simulink model "FinalProject"  (R2023b)
settings: Solver=VariableStepAuto  StartTime=0.0  StopTime=inf  RelTol=1e-3
libraries: instrumentseriallib x3
settings Model: Creator=Ngsanchong  LastModifiedBy=Ngsanchong

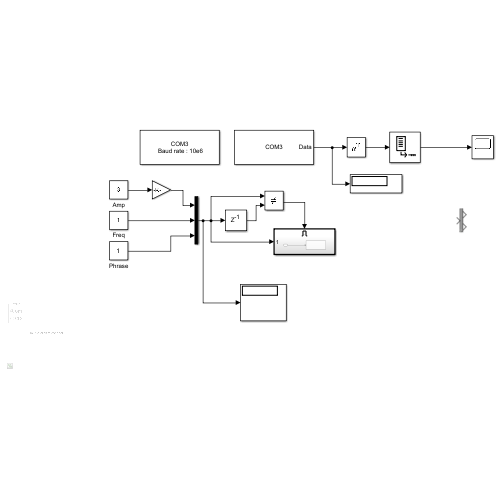
[thumbnail: Simulink's stored preview of the top-level diagram]
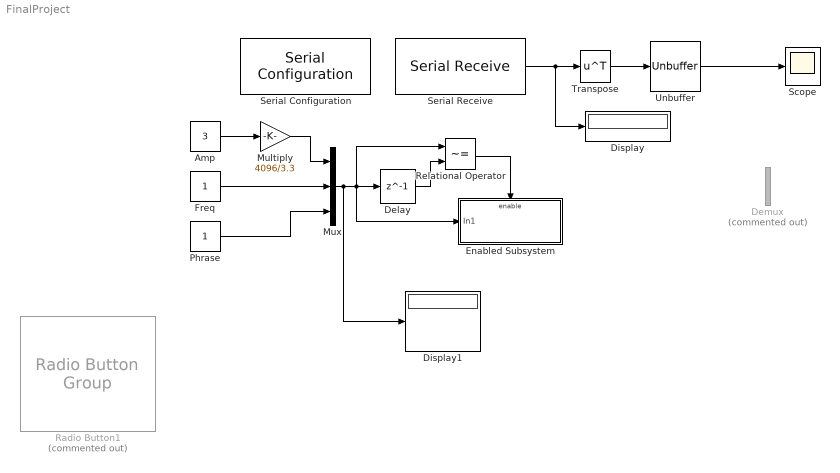
== system FinalProject ==
  Amp : Constant  Value=3  OutDataTypeStr=double
  Delay : Delay  DelayLength=1
  Demux : Demux  Commented=on  Outputs=2
  Display : Display
  Display1 : Display
  Enabled Subsystem : Subsystem  TreatAsAtomicUnit=on
  Freq : Constant  OutDataTypeStr=uint16
  Multiply : Gain  Gain=4096/3.3  OutMin=[0]  OutMax=[4096]  OutDataTypeStr=uint16
  Mux : Mux  Inputs=3
  Phrase : Constant  OutDataTypeStr=uint16
  Radio Button1 : RadioButtonGroup  Commented=on  ButtonGroupName=Group
      settings: Values={{'Ch1', 'Ch2'}, [0 1]}
  Relational Operator : RelationalOperator  Operator=~=  OutDataTypeStr=boolean  RndMeth=Simplest  InputSameDT=off
  Scope : Scope
  Serial Configuration : instrumentseriallib/Serial Configuration  Priority=-200000  PortSel=COM3  Port=COM3  ComPort=COM3  BaudRate=10e6  DataBits=8  Parity=none  StopBits=1  ByteOrder=little-endian  FlowControl=none  Timeout=10  SimulateUsing=Interpreted execution  BlockInModel=on  aMode=1
      settings: LibrarySourceBlock=c2000lib/Host Communication/Serial Configuration
  Serial Receive : instrumentseriallib/Serial Receive  Priority=1  PortSel=COM3  Port=COM3  ComPort=COM3  DataType=int16  SaveDataType=uint8  ToggleHeader=off  Header=[]  ToggleTerminator=off  Terminator=<none>  CustomTerminator=[]  InputFormat=Column major  ToggleDataSize=on  DataSize=[1 2000]  EnableBlockingMode=on  ActionDataUnavailable=Output last received value  ActionWhenDataUnavailable=Output last received value  CustomValue=0  SampleTime=0.02  SimulateUsing=Interpreted execution  BlockInModel=on  aMode=1
      settings: LibrarySourceBlock=c2000lib/Host Communication/Serial Receive
  Transpose : Math  Operator=transpose
  Unbuffer : Unbuffer
  wires:
  Serial Receive/1 -> Display/1, Transpose/1
  Transpose/1 -> Unbuffer/1
  Relational Operator/1 -> Enabled Subsystem/Enable
  Delay/1 -> Relational Operator/2
  Freq/1 -> Mux/2
  Mux/1 -> Display1/1, Enabled Subsystem/1(In1), Relational Operator/1, Delay/1
  Phrase/1 -> Mux/3
  Amp/1 -> Multiply/1
  Multiply/1 -> Mux/1
  Unbuffer/1 -> Scope/1

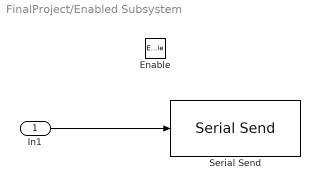
== system FinalProject/Enabled Subsystem ==
  In1 : Inport
  Enable : EnablePort
  Serial Send : instrumentseriallib/Serial Send  Priority=1  PortSel=COM3  Port=COM3  ComPort=COM3  Header=[]  Terminator=<none>  CustomTerminator=[]  EnableBlockingMode=on  SimulateUsing=Interpreted execution  BlockInModel=on  aMode=1
      settings: LibrarySourceBlock=c2000lib/Host Communication/Serial Send
  wires:
  In1/1 -> Serial Send/1
